simulink model "fm"  (R2013b)
settings: Solver=ode45  StartTime=0.0  StopTime=10.0  RelTol=1e-3
libraries: dspsrcs4 x1
settings Model: Creator=Ali  LastModifiedBy=Ali

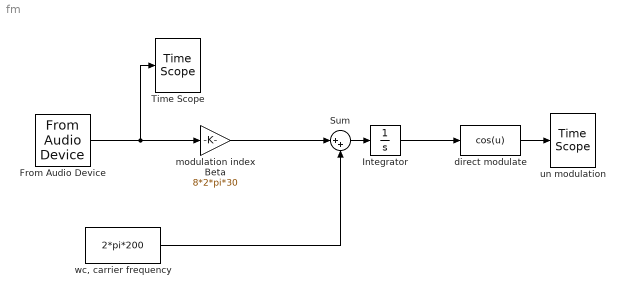
== system fm ==
  From Audio Device : dspsrcs4/From Audio Device  deviceName=Primary Sound Capture Driver  numChannels=1  sampleRate=1200  deviceDatatype=Determine from output data type  autoBufferSize=on  bufferSize=4096  queueDuration=5  frameSize=1  outputDatatype=single  defaultInputChannelMapping=on  inputChannelMapping=1:2
  Integrator : Integrator  IgnoreLimit=on
  Sum : Sum  Inputs=|++
  Time Scope : TimeScope  DefaultConfigurationName=spbscopes.TimeScopeBlockCfg
      settings: CopyFcn=scopeextensions.ScopeBlock.onCoreBlockCopy(gcbh);  DeleteFcn=scopeextensions.ScopeBlock.callback(gcbh, 'onBlockDelete');  PreSaveFcn=scopeextensions.ScopeBlock.callback(gcbh, 'onModelSave');  NameChangeFcn=scopeextensions.ScopeBlock.callback(gcbh, 'onBlockRename');  DestroyFcn=scopeextensions.ScopeBlock.onBlockDestroy(gcbh)  CloseFcn=scopeextensions.ScopeBlock.callback(gcbh, 'onBlockClose');  PreDeleteFcn=scopeextensions.ScopeBlock.callback(gcbh, 'onBlockPreDelete');
  direct modulate : Fcn  Expr=cos(u)
  modulation index Beta : Gain  Gain=8*2*pi*30
  un modulation : TimeScope  DefaultConfigurationName=spbscopes.TimeScopeBlockCfg
      settings: CopyFcn=scopeextensions.ScopeBlock.onCoreBlockCopy(gcbh);  DeleteFcn=scopeextensions.ScopeBlock.callback(gcbh, 'onBlockDelete');  PreSaveFcn=scopeextensions.ScopeBlock.callback(gcbh, 'onModelSave');  NameChangeFcn=scopeextensions.ScopeBlock.callback(gcbh, 'onBlockRename');  DestroyFcn=scopeextensions.ScopeBlock.onBlockDestroy(gcbh)  CloseFcn=scopeextensions.ScopeBlock.callback(gcbh, 'onBlockClose');  PreDeleteFcn=scopeextensions.ScopeBlock.callback(gcbh, 'onBlockPreDelete');
  "wc, carrier frequency" : Constant  Value=2*pi*200
  wires:
  "wc, carrier frequency"/1 -> Sum/2
  Integrator/1 -> direct modulate/1
  direct modulate/1 -> un modulation/1
  Sum/1 -> Integrator/1
  modulation index Beta/1 -> Sum/1
  From Audio Device/1 -> modulation index Beta/1, Time Scope/1
